simulink model "input_generation"  (R2025b)
settings: Solver=VariableStepAuto  StartTime=0.0  StopTime=10.0  RelTol=1e-3
values from neighbouring files (symbols this model uses):
  s_input = struct    [specs_and_input.m]
undefined symbols (not defined in the file or in its folder): Ts
libraries: simulink x1
settings Model: Creator=elia  LastModifiedBy=elia

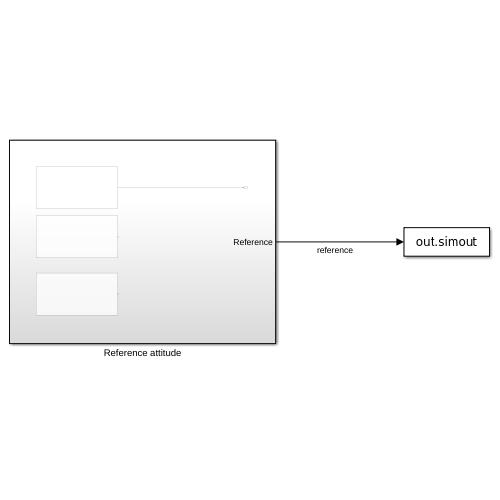
[thumbnail: Simulink's stored preview of the top-level diagram]
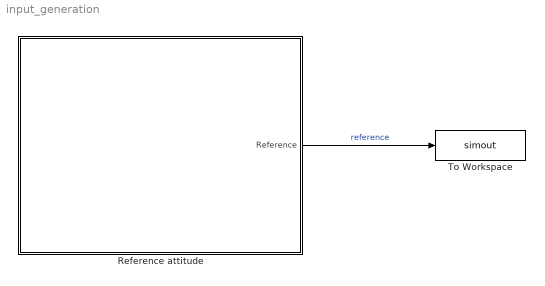
== system input_generation ==
  Reference attitude : Subsystem
  To Workspace : ToWorkspace  VariableName=simout  SaveFormat=Timeseries  SampleTime=-1
  wires:
  Reference attitude/1(Reference) -> To Workspace/1  "reference"

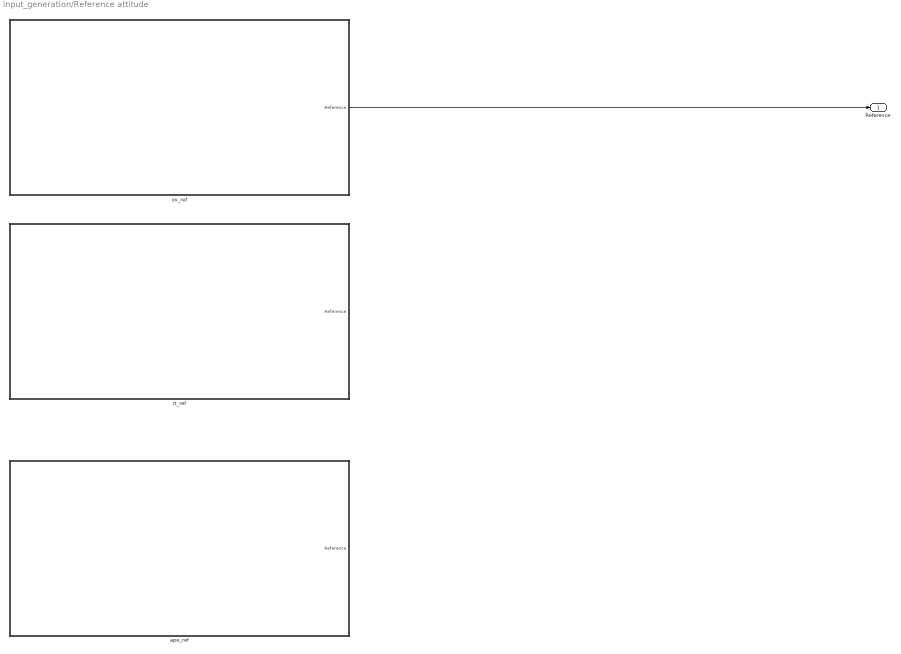
== system input_generation/Reference attitude ==
  ape_ref : Subsystem
  ov_ref : Subsystem
  rt_ref : Subsystem
  Reference : Outport
  wires:
  ov_ref/1(Reference) -> Reference/1

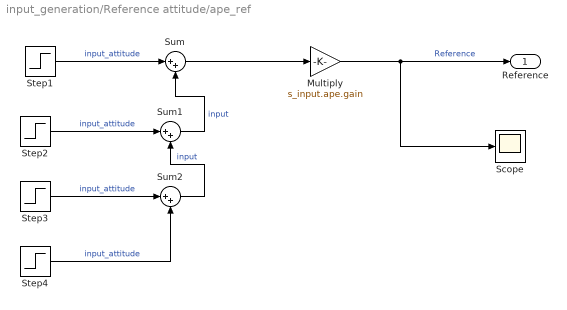
== system input_generation/Reference attitude/ape_ref ==
  Multiply : Gain  Gain=s_input.ape.gain
  Scope : Scope
      settings: ActiveDisplayYMinimum=-1  ActiveDisplayYMaximum=1  DataLoggingVariableName=ScopeData4
  Step1 : Step  Time=s_input.ape.step_1.time  After=s_input.ape.step_1.size  SampleTime=Ts
  Step2 : Step  Time=s_input.ape.step_2.time  After=s_input.ape.step_2.size  SampleTime=Ts
  Step3 : Step  Time=s_input.ape.step_3.time  After=s_input.ape.step_3.size  SampleTime=Ts
  Step4 : Step  Time=s_input.ape.step_4.time  After=s_input.ape.step_4.size  SampleTime=Ts
  Sum : Sum  Inputs=|++
  Sum1 : Sum  Inputs=|++
  Sum2 : Sum  Inputs=|++
  Reference : Outport
  wires:
  Step4/1 -> Sum2/2  "input_attitude"
  Step3/1 -> Sum2/1  "input_attitude"
  Multiply/1 -> Reference/1, Scope/1  "Reference"
  Step2/1 -> Sum1/1  "input_attitude"
  Step1/1 -> Sum/1  "input_attitude"
  Sum1/1 -> Sum/2  "input"
  Sum2/1 -> Sum1/2  "input"
  Sum/1 -> Multiply/1

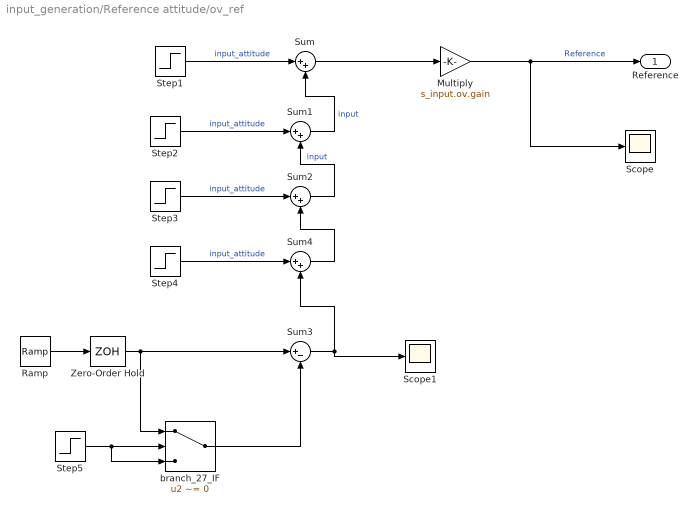
== system input_generation/Reference attitude/ov_ref ==
  Multiply : Gain  Gain=s_input.ov.gain
  Ramp : simulink/Sources/Ramp  slope=1  start=6  InitialOutput=0
  Scope : Scope
      settings: ActiveDisplayYMinimum=-31.173012433294765  ActiveDisplayYMaximum=78.275517903912672  DataLoggingVariableName=ScopeData4
  Scope1 : Scope
      settings: ActiveDisplayYMinimum=-11.656452979221982  ActiveDisplayYMaximum=31.656047020778054  DataLoggingVariableName=ScopeData6
  Step1 : Step  Time=s_input.ov.step_1.time  After=s_input.ov.step_1.size  SampleTime=Ts
  Step2 : Step  Time=s_input.ov.step_2.time  After=s_input.ov.step_2.size  SampleTime=Ts
  Step3 : Step  Time=s_input.ov.step_3.time  After=s_input.ov.step_3.size  SampleTime=Ts
  Step4 : Step  Time=s_input.ov.step_4.time  After=s_input.ov.step_4.size  SampleTime=Ts
  Step5 : Step  Time=8.5  SampleTime=Ts
  Sum{,1..2,4} (4 alike) : Sum  Inputs=|++
  Sum3 : Sum  Inputs=|+-
  Zero-Order Hold : ZeroOrderHold  SampleTime=Ts
  branch_27_IF : Switch  Criteria=u2 ~= 0  SaturateOnIntegerOverflow=off  InputSameDT=off
  Reference : Outport
  wires:
  Step4/1 -> Sum4/1  "input_attitude"
  Step3/1 -> Sum2/1  "input_attitude"
  Multiply/1 -> Reference/1, Scope/1  "Reference"
  Step2/1 -> Sum1/1  "input_attitude"
  Step1/1 -> Sum/1  "input_attitude"
  Sum1/1 -> Sum/2  "input"
  Sum2/1 -> Sum1/2  "input"
  Sum/1 -> Multiply/1
  Ramp/1 -> Zero-Order Hold/1
  Sum4/1 -> Sum2/2
  Sum3/1 -> Scope1/1, Sum4/2
  Zero-Order Hold/1 -> branch_27_IF/1, Sum3/1
  branch_27_IF/1 -> Sum3/2
  Step5/1 -> branch_27_IF/2, branch_27_IF/3

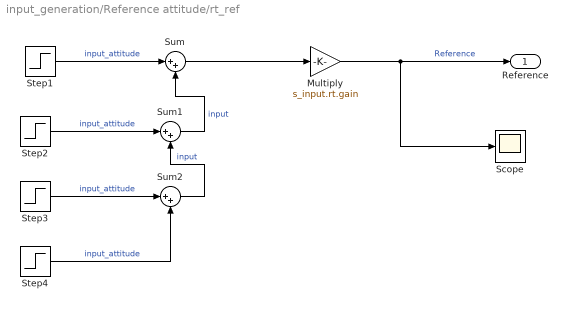
== system input_generation/Reference attitude/rt_ref ==
  Multiply : Gain  Gain=s_input.rt.gain
  Scope : Scope
      settings: ActiveDisplayYMinimum=-1  ActiveDisplayYMaximum=1  DataLoggingVariableName=ScopeData4
  Step1 : Step  Time=s_input.rt.step_1.time  After=s_input.rt.step_1.size  SampleTime=Ts
  Step2 : Step  Time=s_input.rt.step_2.time  After=s_input.rt.step_2.size  SampleTime=Ts
  Step3 : Step  Time=s_input.rt.step_3.time  After=s_input.rt.step_3.size  SampleTime=Ts
  Step4 : Step  Time=s_input.rt.step_4.time  After=s_input.rt.step_4.size  SampleTime=Ts
  Sum : Sum  Inputs=|++
  Sum1 : Sum  Inputs=|++
  Sum2 : Sum  Inputs=|++
  Reference : Outport
  wires:
  Step4/1 -> Sum2/2  "input_attitude"
  Step3/1 -> Sum2/1  "input_attitude"
  Multiply/1 -> Reference/1, Scope/1  "Reference"
  Step2/1 -> Sum1/1  "input_attitude"
  Step1/1 -> Sum/1  "input_attitude"
  Sum1/1 -> Sum/2  "input"
  Sum2/1 -> Sum1/2  "input"
  Sum/1 -> Multiply/1
